simulink model "untitled2"  (R2023b)
settings: Solver=VariableStepAuto  StartTime=0.0  StopTime=10  RelTol=1e-3
libraries: dspfdesign x2, dspsigops x1, spspowerguiLib x1
settings Model: Creator=mrabd  LastModifiedBy=mrabd

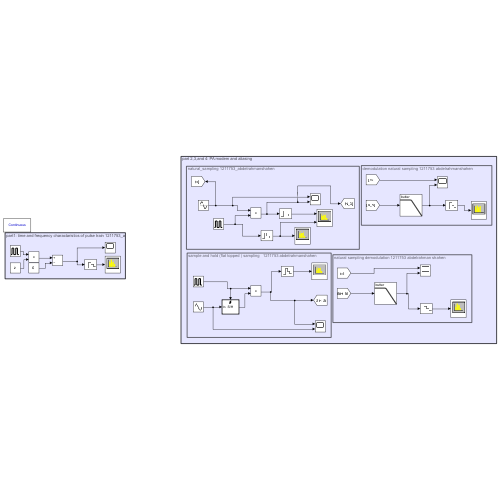
[thumbnail: Simulink's stored preview of the top-level diagram]
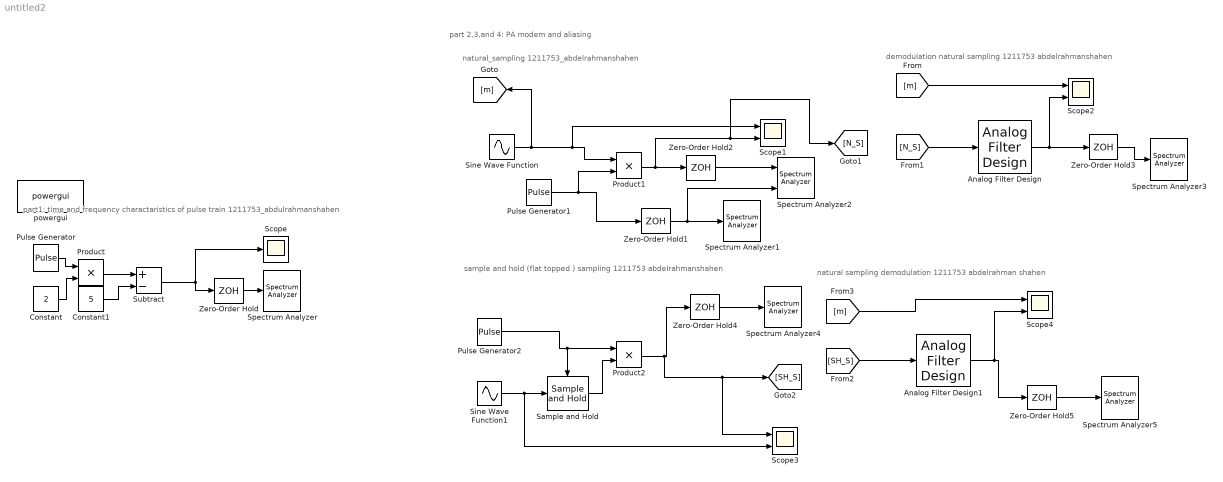
== system untitled2 ==
  note: part 2,3,and 4: PA modem and aliasing
  note: part1: time and frequency charactaristics of pulse train 1211753_abdulrahmanshahen
  note: natural_sampling 1211753_abdelrahmanshahen
  note: demodulation natural sampling 1211753 abdelrahmanshahen
  note: sample and hold (flat topped ) sampling 1211753 abdelrahmanshahen
  note: natural sampling demodulation 1211753 abdelrahman shahen
  Analog Filter Design : dspfdesign/Analog Filter Design  method=Butterworth  filttype=Lowpass  N=8  Wlo=3400  Whi=80  Rp=2  Rs=40
  Analog Filter Design1 : dspfdesign/Analog Filter Design  method=Butterworth  filttype=Lowpass  N=8  Wlo=3400  Whi=80  Rp=2  Rs=40
  Constant : Constant  Value=2
  Constant1 : Constant  Value=5
  Product : Product
  Product1 : Product
  Product2 : Product
  Pulse Generator : DiscretePulseGenerator  PulseType=Time based  Amplitude=10  Period=1/1000  PulseWidth=10
  Pulse Generator1 : DiscretePulseGenerator  PulseType=Time based  Amplitude=10  Period=1/1000  PulseWidth=10
  Pulse Generator2 : DiscretePulseGenerator  PulseType=Time based  Amplitude=10  Period=1/1000  PulseWidth=10
  Sample and Hold : dspsigops/Sample and Hold  trig=Rising edge  initCond=0  latchinput=off
  Scope : Scope
  Scope{1..4} (4 alike) : Scope  NumInputPorts=2
  Sine Wave Function : Sin  Amplitude=10  Frequency=1000  SampleTime=0
  Sine Wave Function1 : Sin  Amplitude=10  Frequency=1000  SampleTime=0
  Spectrum Analyzer : SpectrumAnalyzer  WindowPosition=[1.000000,41.000000,1536.000000,801.000000,]  ScopeFrameLocation=window  SampleRateSource=Property  SampleRate=44.1e3  PlotAsTwoSidedSpectrum=off  FrequencyScale=Log  FrequencySpan=Start and stop frequencies  StartFrequency=20  StopFrequency=20e3  YLimits=[-139.75407289,-50.47835773]
  Spectrum Analyzer1 : SpectrumAnalyzer  WindowPosition=[368.000000,217.000000,800.000000,501.000000,]  ScopeFrameLocation=window  SampleRateSource=Property  SampleRate=44.1e3  PlotAsTwoSidedSpectrum=off  FrequencyScale=Log  FrequencySpan=Start and stop frequencies  StartFrequency=20  StopFrequency=20e3  YLimits=[-451.81505353,-448.05217859]
  Spectrum Analyzer2 : SpectrumAnalyzer  NumInputPorts=2  WindowPosition=[1.000000,41.000000,1536.000000,801.000000,]  ScopeFrameLocation=window  SampleRateSource=Property  SampleRate=44.1e3  PlotAsTwoSidedSpectrum=off  FrequencyScale=Log  FrequencySpan=Start and stop frequencies  StartFrequency=20  StopFrequency=20e3  YLimits=[-147.32924315,-41.6495873]
  Spectrum Analyzer3 : SpectrumAnalyzer  WindowPosition=[1.000000,41.000000,1536.000000,801.000000,]  ScopeFrameLocation=window  SampleRateSource=Property  SampleRate=44.1e3  PlotAsTwoSidedSpectrum=off  FrequencyScale=Log  FrequencySpan=Start and stop frequencies  StartFrequency=20  StopFrequency=20e3  YLimits=[-186.96943253,-37.23589219]
  Spectrum Analyzer4 : SpectrumAnalyzer  WindowPosition=[1.000000,41.000000,1536.000000,801.000000,]  ScopeFrameLocation=window  SampleRateSource=Property  SampleRate=44.1e3  PlotAsTwoSidedSpectrum=off  FrequencyScale=Log  FrequencySpan=Start and stop frequencies  StartFrequency=20  StopFrequency=20e3  YLimits=[-135.30752035,-42.9877843]
  Spectrum Analyzer5 : SpectrumAnalyzer  WindowPosition=[1.000000,41.000000,1536.000000,801.000000,]  ScopeFrameLocation=window  SampleRateSource=Property  SampleRate=44.1e3  PlotAsTwoSidedSpectrum=off  FrequencyScale=Log  FrequencySpan=Start and stop frequencies  StartFrequency=20  StopFrequency=20e3  YLimits=[-188.47202844,-37.07295706]
  Subtract : Sum  Inputs=+-
  Zero-Order Hold{,1..5} (6 alike) : ZeroOrderHold  SampleTime=-1
  powergui : spspowerguiLib/powergui  Priority=1  SimulationMode=Continuous  SampleTime=50e-6  frequency=60  Iterations=50  frequencyindice=60  Pbase=100e6  ErrMax=1e-4  UnitsV=kV  UnitsW=MW  buscounter=0  FunctionMessages=off  echomessages=off  EnableUseOfTLC=off  CurrentSourceSwitches=off  DisableSnubberDevices=off  DisableRonSwitches=off  DisableVfSwitches=off  DisplayEquations=off  AutomaticDiscreteSolvers=off  SolverType=Tustin/Backward Euler (TBE)  Interpol=off  ExternalGateDelay=off  methode=off  Ts=100  x0status=blocks  SPID=on  SwTol=0  HookPort=off  NonlinearTolerance=1e-4  nMaxIteration=100  ContinueOnMaxIteration=off  RestoreLinks=warning  ResistiveCurrentMeasurement=off  Frange=[0:2:500]  Ylog=off  Xlog=on  ShowGrid=off  save=off  variable=ZData  structure=0  ZoomFFT=off  StartTime=0.0  cycles=1  DisplayStyle=1  fundamental=60  FreqAxis=off  MaxFrequency=1000  frequencyindicesteady=1  RmsSteady=1  display=off
  wires:
  Pulse Generator/1 -> Product/1
  Product/1 -> Subtract/1
  Constant/1 -> Product/2
  Zero-Order Hold/1 -> Spectrum Analyzer/1
  Constant1/1 -> Subtract/2
  Subtract/1 -> Zero-Order Hold/1, Scope/1
  [SH_S] -> Analog Filter Design1/1
  [m] -> Scope4/1
  [N_S] -> Analog Filter Design/1
  [m] -> Scope2/1
  Zero-Order Hold3/1 -> Spectrum Analyzer3/1
  Sine Wave Function1/1 -> Scope3/2, Sample and Hold/1
  Analog Filter Design1/1 -> Scope4/2, Zero-Order Hold5/1
  Zero-Order Hold5/1 -> Spectrum Analyzer5/1
  Sine Wave Function/1 -> [m], Scope1/1, Product1/1
  Analog Filter Design/1 -> Scope2/2, Zero-Order Hold3/1
  Sample and Hold/1 -> Product2/2
  Pulse Generator2/1 -> Sample and Hold/Trigger, Product2/1
  Zero-Order Hold4/1 -> Spectrum Analyzer4/1
  Pulse Generator1/1 -> Product1/2, Zero-Order Hold1/1
  Zero-Order Hold1/1 -> Spectrum Analyzer2/2, Spectrum Analyzer1/1
  Product2/1 -> Scope3/1, [SH_S], Zero-Order Hold4/1
  Product1/1 -> [N_S], Scope1/2, Zero-Order Hold2/1
  Zero-Order Hold2/1 -> Spectrum Analyzer2/1
